simulink model "blinkchallenge"  (Simulink 7.4)
settings: Solver=ode45  StartTime=0.0  StopTime=10.0  RelTol=1e-3
libraries: elec_lib x15, fl_lib x11
settings Model: Creator=gcampa  LastModifiedBy=gcampa

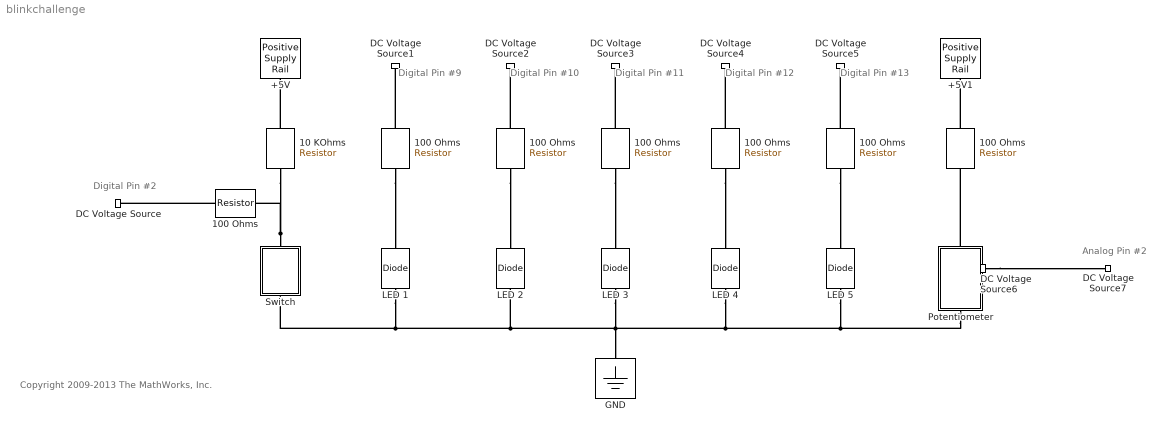
== system blinkchallenge ==
  note: Digital Pin #2
  note: Digital
      | Pin #9
  note: Digital
      | Pin #10
  note: Digital
      | Pin #11
  note: Digital
      | Pin #12
  note: Digital
      | Pin #13
  note: Analog Pin #2
  note: Copyright 2009-2013 The MathWorks, Inc.
  "  Potentiometer" : Subsystem
      mask Display:
      | plot([45.5890141893179;79.6036154497415;90.9418158698828;113.618216710165;136.294617550448;158.97101839073;181.647419231013;204.323820071295;227.000220911577;249.67662175186;261.014822172001;295.029423432425], 28.10+[85.2727156598121;85.2727156598121;107.949116500095;62.5963148195297;107.949116500095;62.5963148195297;107.949116500095;62.5963148195297;107.949116500095;62.5963148195297;85.2727156598121;85.2727156598121])
      | plot([0.236212508752999;45.5890141893179;45.5890141893179], 28.10+[85.2727156598121;85.2727156598121;85.2727156598121])
      | plot([295.029423432425;295.029423432425;340.38222511299], 28.10+[85.2727156598121;85.2727156598121;85.2727156598121])
      | plot([109.280016290024;109.280016290024;124.956417130306;232.669321121648], 28.10+[210.309218810871;170.309218810871;141.963717760518;20.0780632440001])
      | plot([209.992920281366;232.669321121648;232.669321121648], 28.10+[20.0780632440001;20.0780632440001;42.7544640842825])
      | patch([5.6843418860808e-14;340.618437621743;340.618437621743;0;5.6843418860808e-14;0.472425017505941;0.472425017505941;340.146012604237;340.146012604237;0.472425017505941;5.6843418860808e-14], [227.23643342033;227.23643342033;0;0;227.23643342033;226.764008402824;0.472425017505884;0.472425017505884;226.764008402824;226.764008402824;227.23643342033], [1;1;1]);
  +5V : elec_lib/Sources/Positive Supply Rail  DialogController=NetworkEngine.DynNeDlgSource  SystemSampleTime=-1  v0=1 V  current_Log=off  voltage_Log=off  power_Log=off  LocalVarNames=|current|voltage|power  LocalVarDescs=|Current (A)|Voltage (V)|Power (W)  LocalVarLogging=[0 0 0]
  +5V1 : elec_lib/Sources/Positive Supply Rail  DialogController=NetworkEngine.DynNeDlgSource  SystemSampleTime=-1  v0=1 V  current_Log=off  voltage_Log=off  power_Log=off  LocalVarNames=|current|voltage|power  LocalVarDescs=|Current (A)|Voltage (V)|Power (W)  LocalVarLogging=[0 0 0]
  10 KOhms : elec_lib/Passive Devices/Resistor  DialogController=NetworkEngine.DynNeDlgSource  SystemSampleTime=-1  SCALE=1  R_param=1  R=0 Ohm  RSH=0 Ohm  LENGTH=1e-06 m  WIDTH=1e-06 m  NARROW=0 m  T_param=1  TC1=0 1/K  TC2=0 1/K^2  TOFFSET=0 K  TFIXED=300.15 K  TMEAS=300.15 K  LocalVarLogging=[]
  100 Ohms : elec_lib/Passive Devices/Resistor  DialogController=NetworkEngine.DynNeDlgSource  SystemSampleTime=-1  SCALE=1  R_param=1  R=0 Ohm  RSH=0 Ohm  LENGTH=1e-06 m  WIDTH=1e-06 m  NARROW=0 m  T_param=1  TC1=0 1/K  TC2=0 1/K^2  TOFFSET=0 K  TFIXED=300.15 K  TMEAS=300.15 K  LocalVarLogging=[]
  "100 Ohms         " : elec_lib/Passive Devices/Resistor  DialogController=NetworkEngine.DynNeDlgSource  SystemSampleTime=-1  SCALE=1  R_param=1  R=0 Ohm  RSH=0 Ohm  LENGTH=1e-06 m  WIDTH=1e-06 m  NARROW=0 m  T_param=1  TC1=0 1/K  TC2=0 1/K^2  TOFFSET=0 K  TFIXED=300.15 K  TMEAS=300.15 K  LocalVarLogging=[]
  "100 Ohms " : elec_lib/Passive Devices/Resistor  DialogController=NetworkEngine.DynNeDlgSource  SystemSampleTime=-1  SCALE=1  R_param=1  R=0 Ohm  RSH=0 Ohm  LENGTH=1e-06 m  WIDTH=1e-06 m  NARROW=0 m  T_param=1  TC1=0 1/K  TC2=0 1/K^2  TOFFSET=0 K  TFIXED=300.15 K  TMEAS=300.15 K  LocalVarLogging=[]
  "100 Ohms  " : elec_lib/Passive Devices/Resistor  DialogController=NetworkEngine.DynNeDlgSource  SystemSampleTime=-1  SCALE=1  R_param=1  R=0 Ohm  RSH=0 Ohm  LENGTH=1e-06 m  WIDTH=1e-06 m  NARROW=0 m  T_param=1  TC1=0 1/K  TC2=0 1/K^2  TOFFSET=0 K  TFIXED=300.15 K  TMEAS=300.15 K  LocalVarLogging=[]
  "100 Ohms   " : elec_lib/Passive Devices/Resistor  DialogController=NetworkEngine.DynNeDlgSource  SystemSampleTime=-1  SCALE=1  R_param=1  R=0 Ohm  RSH=0 Ohm  LENGTH=1e-06 m  WIDTH=1e-06 m  NARROW=0 m  T_param=1  TC1=0 1/K  TC2=0 1/K^2  TOFFSET=0 K  TFIXED=300.15 K  TMEAS=300.15 K  LocalVarLogging=[]
  "100 Ohms    " : elec_lib/Passive Devices/Resistor  DialogController=NetworkEngine.DynNeDlgSource  SystemSampleTime=-1  SCALE=1  R_param=1  R=0 Ohm  RSH=0 Ohm  LENGTH=1e-06 m  WIDTH=1e-06 m  NARROW=0 m  T_param=1  TC1=0 1/K  TC2=0 1/K^2  TOFFSET=0 K  TFIXED=300.15 K  TMEAS=300.15 K  LocalVarLogging=[]
  "100 Ohms          " : elec_lib/Passive Devices/Resistor  DialogController=NetworkEngine.DynNeDlgSource  SystemSampleTime=-1  SCALE=1  R_param=1  R=0 Ohm  RSH=0 Ohm  LENGTH=1e-06 m  WIDTH=1e-06 m  NARROW=0 m  T_param=1  TC1=0 1/K  TC2=0 1/K^2  TOFFSET=0 K  TFIXED=300.15 K  TMEAS=300.15 K  LocalVarLogging=[]
  DC Voltage Source{,1..7} (8 alike) : fl_lib/Electrical/Electrical Sources/DC Voltage Source  DialogController=NetworkEngine.DynNeDlgSource  SystemSampleTime=-1  v0=1 V  i_Log=off  v_Log=off  LocalVarNames=|i|v  LocalVarDescs=|i|v  LocalVarLogging=[0 0]
  GND : fl_lib/Electrical/Electrical Elements/Electrical Reference  DialogController=NetworkEngine.DynNeDlgSource  SystemSampleTime=-1  i_Log=off  LocalVarNames=|i  LocalVarDescs=|i  LocalVarLogging=0
  LED {1..5} (5 alike) : elec_lib/Semiconductor Devices/Diode  DialogController=NetworkEngine.DynNeDlgSource  SystemSampleTime=-1  ModelType=1  Vf=0.6 V  Ron=0.3 Ohm  Goff=1e-08 S  Rz=0.3 Ohm  Vz=50 V  C_PWL=5 pF  prmExp=1  I12="[  0.07 1.5 ] A"  V12="[  0.7 0.8 ] V"  RS=0.01 Ohm  IS=1e-14 A  Tmeas=25 C  ec=1  BV=Inf V  C_param=1  CJ0=5 pF  VJ=1 V  Mgrad=0.5  Vvec="[  0.1 10 100 ] V"  Cvec="[  3.5 1 0.4 ] pF"  FC=0.5  LocalVarLogging=[]
  Switch : Subsystem
      mask Display:
      | patch([178.308949107304;178.270428219378;178.155236532808;177.964483406507;177.700005897356;177.364351068347;176.960751458971;176.493093954097;175.965882351142;175.384193986049;174.753630835755;174.080265568098;173.370583058705;172.631417938094;171.869888770445;171.093329497935;170.309218810871;169.525108123807;168.748548851298;167.987019683648;167.247854563037;166.538172053645;165.864806785988;165.234243635694;164.6525552706;164.125343667646;163.657686162771;163.254086553395;162.918431724386;162.653954215236;162.463201088934;162.348009402364;162.309488514438;162.348009402364;162.463201088934;162.653954215236;162.918431724386;163.254086553395;163.657686162771;164.125343667646;164.6525552706;165.234243635694;165.864806785988;166.538172053645;167.247854563037;167.987019683648;168.748548851298;169.525108123807;170.309218810871;171.093329497935;171.869888770445;172.631417938094;173.370583058705;174.080265568098;174.753630835754;175.384193986049;175.965882351142;176.493093954096;176.960751458971;177.364351068347;177.700005897356;177.964483406507;178.155236532808;178.270428219378;178.308949107304;178.308949107304], [113.618216710165;112.834106023101;112.057546750592;111.296017582942;110.556852462331;109.847169952939;109.173804685282;108.543241534988;107.961553169894;107.43434156694;106.966684062065;106.563084452689;106.22742962368;105.962952114529;105.772198988228;105.657007301658;105.618486413732;105.657007301658;105.772198988228;105.962952114529;106.22742962368;106.563084452689;106.966684062065;107.43434156694;107.961553169894;108.543241534988;109.173804685282;109.847169952939;110.556852462331;111.296017582942;112.057546750592;112.834106023101;113.618216710165;114.402327397229;115.178886669738;115.940415837388;116.679580957999;117.389263467392;118.062628735048;118.693191885343;119.274880250436;119.80209185339;120.269749358265;120.673348967641;121.00900379665;121.273481305801;121.464234432102;121.579426118672;121.617947006598;121.579426118672;121.464234432102;121.273481305801;121.00900379665;120.673348967641;120.269749358265;119.80209185339;119.274880250436;118.693191885343;118.062628735048;117.389263467392;116.679580957999;115.940415837388;115.178886669738;114.402327397229;113.618216710165;113.618216710165], [0;0;0])
      | plot([178.308949107304;178.270428219378;178.155236532808;177.964483406507;177.700005897356;177.364351068347;176.960751458971;176.493093954097;175.965882351142;175.384193986049;174.753630835755;174.080265568098;173.370583058705;172.631417938094;171.869888770445;171.093329497935;170.309218810871;169.525108123807;168.748548851298;167.987019683648;167.247854563037;166.538172053645;165.864806785988;165.234243635694;164.6525552706;164.125343667646;163.657686162771;163.254086553395;162.918431724386;162.653954215236;162.463201088934;162.348009402364;162.309488514438;162.348009402364;162.463201088934;162.653954215236;162.918431724386;163.254086553395;163.657686162771;164.125343667646;164.6525552706;165.234243635694;165.864806785988;166.538172053645;167.247854563037;167.987019683648;168.748548851298;169.525108123807;170.309218810871;171.093329497935;171.869888770445;172.631417938094;173.370583058705;174.080265568098;174.753630835754;175.384193986049;175.965882351142;176.493093954096;176.960751458971;177.364351068347;177.700005897356;177.964483406507;178.155236532808;178.270428219378;178.308949107304;178.308949107304], [113.618216710165;112.834106023101;112.057546750592;111.296017582942;110.556852462331;109.847169952939;109.173804685282;108.543241534988;107.961553169894;107.43434156694;106.966684062065;106.563084452689;106.22742962368;105.962952114529;105.772198988228;105.657007301658;105.618486413732;105.657007301658;105.772198988228;105.962952114529;106.22742962368;106.563084452689;106.966684062065;107.43434156694;107.961553169894;108.543241534988;109.173804685282;109.847169952939;110.556852462331;111.296017582942;112.057546750592;112.834106023101;113.618216710165;114.402327397229;115.178886669738;115.940415837388;116.679580957999;117.389263467392;118.062628735048;118.693191885343;119.274880250436;119.80209185339;120.269749358265;120.673348967641;121.00900379665;121.273481305801;121.464234432102;121.579426118672;121.617947006598;121.579426118672;121.464234432102;121.273481305801;121.00900379665;120.673348967641;120.269749358265;119.80209185339;119.274880250436;118.693191885343;118.062628735048;117.389263467392;116.679580957999;115.940415837388;115.178886669738;114.402327397229;113.618216710165;113.618216710165])
      | patch([64.926944905892;64.888424017966;64.7732323313963;64.5824792050947;64.3180016959439;63.9823468669351;63.5787472575591;63.1110897526843;62.5838781497303;62.0021897846366;61.3716266343423;60.6982613666856;59.988578857293;59.2494137366818;58.4878845690323;57.7113252965232;56.927214609459;56.1431039223949;55.3665446498857;54.6050154822362;53.8658503616251;53.1561678522324;52.4828025845758;51.8522394342815;51.2705510691878;50.7433394662337;50.275681961359;49.872082351983;49.5364275229742;49.2719500138234;49.0811968875218;48.9660052009521;48.9274843130261;48.9660052009521;49.0811968875218;49.2719500138234;49.5364275229742;49.8720823519831;50.275681961359;50.7433394662338;51.2705510691878;51.8522394342816;52.4828025845758;53.1561678522325;53.8658503616251;54.6050154822362;55.3665446498858;56.143103922395;56.927214609459;57.7113252965232;58.4878845690323;59.2494137366818;59.988578857293;60.6982613666856;61.3716266343422;62.0021897846366;62.5838781497303;63.1110897526843;63.5787472575591;63.982346866935;64.3180016959439;64.5824792050947;64.7732323313963;64.888424017966;64.926944905892;64.926944905892], [113.618216710165;112.834106023101;112.057546750592;111.296017582942;110.556852462331;109.847169952939;109.173804685282;108.543241534988;107.961553169894;107.43434156694;106.966684062065;106.563084452689;106.22742962368;105.962952114529;105.772198988228;105.657007301658;105.618486413732;105.657007301658;105.772198988228;105.962952114529;106.22742962368;106.563084452689;106.966684062065;107.43434156694;107.961553169894;108.543241534988;109.173804685282;109.847169952939;110.556852462331;111.296017582942;112.057546750592;112.834106023101;113.618216710165;114.402327397229;115.178886669738;115.940415837388;116.679580957999;117.389263467392;118.062628735048;118.693191885343;119.274880250436;119.80209185339;120.269749358265;120.673348967641;121.00900379665;121.273481305801;121.464234432102;121.579426118672;121.617947006598;121.579426118672;121.464234432102;121.273481305801;121.00900379665;120.673348967641;120.269749358265;119.80209185339;119.274880250436;118.693191885343;118.062628735048;117.389263467392;116.679580957999;115.940415837388;115.178886669738;114.402327397229;113.618216710165;113.618216710165], [0;0;0])
      | plot([64.926944905892;64.888424017966;64.7732323313963;64.5824792050947;64.3180016959439;63.9823468669351;63.5787472575591;63.1110897526843;62.5838781497303;62.0021897846366;61.3716266343423;60.6982613666856;59.988578857293;59.2494137366818;58.4878845690323;57.7113252965232;56.927214609459;56.1431039223949;55.3665446498857;54.6050154822362;53.8658503616251;53.1561678522324;52.4828025845758;51.8522394342815;51.2705510691878;50.7433394662337;50.275681961359;49.872082351983;49.5364275229742;49.2719500138234;49.0811968875218;48.9660052009521;48.9274843130261;48.9660052009521;49.0811968875218;49.2719500138234;49.5364275229742;49.8720823519831;50.275681961359;50.7433394662338;51.2705510691878;51.8522394342816;52.4828025845758;53.1561678522325;53.8658503616251;54.6050154822362;55.3665446498858;56.143103922395;56.927214609459;57.7113252965232;58.4878845690323;59.2494137366818;59.988578857293;60.6982613666856;61.3716266343422;62.0021897846366;62.5838781497303;63.1110897526843;63.5787472575591;63.982346866935;64.3180016959439;64.5824792050947;64.7732323313963;64.888424017966;64.926944905892;64.926944905892], [113.618216710165;112.834106023101;112.057546750592;111.296017582942;110.556852462331;109.847169952939;109.173804685282;108.543241534988;107.961553169894;107.43434156694;106.966684062065;106.563084452689;106.22742962368;105.962952114529;105.772198988228;105.657007301658;105.618486413732;105.657007301658;105.772198988228;105.962952114529;106.22742962368;106.563084452689;106.966684062065;107.43434156694;107.961553169894;108.543241534988;109.173804685282;109.847169952939;110.556852462331;111.296017582942;112.057546750592;112.834106023101;113.618216710165;114.402327397229;115.178886669738;115.940415837388;116.679580957999;117.389263467392;118.062628735048;118.693191885343;119.274880250436;119.80209185339;120.269749358265;120.673348967641;121.00900379665;121.273481305801;121.464234432102;121.579426118672;121.617947006598;121.579426118672;121.464234432102;121.273481305801;121.00900379665;120.673348967641;120.269749358265;119.80209185339;119.274880250436;118.693191885343;118.062628735048;117.389263467392;116.679580957999;115.940415837388;115.178886669738;114.402327397229;113.618216710165;113.618216710165])
      | plot([56.927214609459;161.805568495765], [113.618216710165;56.927214609459])
      | patch([0;227.23643342033;227.23643342033;0;0;0.472425017505884;0.472425017505884;226.764008402824;226.764008402824;0.472425017505884;0], [227.23643342033;227.23643342033;0;0;227.23643342033;226.764008402824;0.472425017505884;0.472425017505884;226.764008402824;226.764008402824;227.23643342033], [1;1;1])
      | plot([170.309218810871;198.654719861224;198.654719861224;227.000220911577], [113.618216710165;113.618216710165;113.618216710165;113.618216710165])
      | plot([56.927214609459;0.236212508752942], [113.618216710165;113.618216710165]);
  connections:
  Switch/RConn1 -- 10 KOhms/RConn1 -- "100 Ohms         "/LConn1
  "100 Ohms         "/RConn1 -- DC Voltage Source/LConn1
  "  Potentiometer"/RConn1 -- LED 5/RConn1 -- LED 3/RConn1 -- LED 2/RConn1 -- LED 1/RConn1 -- Switch/LConn1 -- GND/LConn1 -- LED 4/RConn1
  10 KOhms/LConn1 -- +5V/RConn1
  100 Ohms/RConn1 -- LED 1/LConn1
  100 Ohms/LConn1 -- DC Voltage Source1/RConn1
  "100 Ohms "/RConn1 -- LED 2/LConn1
  "100 Ohms "/LConn1 -- DC Voltage Source2/RConn1
  "100 Ohms  "/LConn1 -- DC Voltage Source3/RConn1
  "100 Ohms  "/RConn1 -- LED 3/LConn1
  "100 Ohms   "/RConn1 -- LED 4/LConn1
  "100 Ohms   "/LConn1 -- DC Voltage Source4/RConn1
  "100 Ohms    "/LConn1 -- DC Voltage Source5/RConn1
  "100 Ohms    "/RConn1 -- LED 5/LConn1
  "  Potentiometer"/LConn1 -- "100 Ohms          "/RConn1
  "100 Ohms          "/LConn1 -- +5V1/RConn1
  DC Voltage Source6/LConn1 -- DC Voltage Source7/RConn1

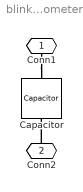
== system blinkchallenge/  Potentiometer ==
  Capacitor : fl_lib/Electrical/Electrical Elements/Capacitor  DialogController=NetworkEngine.DynNeDlgSource  SystemSampleTime=-1  c=1e-06 F  v0=0 V  r=1e-06 Ohm  g=0 1/Ohm  i_Log=off  v_Log=off  vc_Log=off  LocalVarNames=|i|v|vc  LocalVarDescs=|i|v|Internal variable for voltage across capacitor term  LocalVarLogging=[0 0 0]
  Conn1 : PMIOPort  Port=1  Side=Right
  Conn2 : PMIOPort  Port=2  Side=Left
  connections:
  Conn1/RConn1 -- Capacitor/RConn1
  Conn2/RConn1 -- Capacitor/LConn1

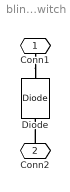
== system blinkchallenge/Switch ==
  Diode : fl_lib/Electrical/Electrical Elements/Diode  DialogController=NetworkEngine.DynNeDlgSource  SystemSampleTime=-1  Vf=0.6 V  Ron=0.3 Ohm  Goff=1e-08 1/Ohm  i_Log=off  v_Log=off  LocalVarNames=|i|v  LocalVarDescs=|i|v  LocalVarLogging=[0 0]
  Conn1 : PMIOPort  Port=1  Side=Right
  Conn2 : PMIOPort  Port=2  Side=Left
  connections:
  Conn1/RConn1 -- Diode/RConn1
  Conn2/RConn1 -- Diode/LConn1
